simulink model "Model4"  (R2018b)
settings: Solver=VariableStepAuto  StartTime=0.0  StopTime=10.0  RelTol=1e-3
values from neighbouring files (symbols this model uses):
  P = 0    [Model.m]
undefined symbols (not defined in the file or in its folder): Ts
settings Model: Creator=Fabi Kadir  LastModifiedBy=Fabi Kadir

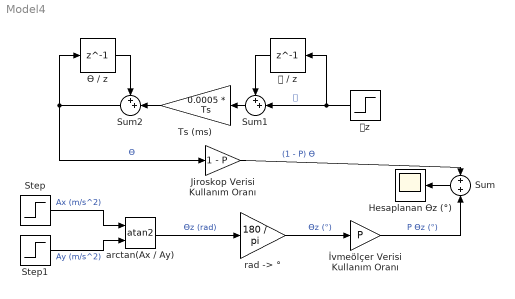
== system Model4 ==
  Hesaplanan Өz (°) : Scope
  Jiroskop Verisi Kullanım Oranı : Gain  Gain=1 - P
  Step : Step  SampleTime=0
  Step1 : Step  SampleTime=0
  Sum : Sum  Inputs=+|+
  Sum1 : Sum  Inputs=++|
  Sum2 : Sum  Inputs=++|
  Ts (ms) : Gain  Gain=0.0005 * Ts
  arctan(Ax / Ay) : Trigonometry  Operator=atan2
  "rad -> °" : Gain  Gain=180 / pi
  İvmeölçer Verisi Kullanım Oranı : Gain  Gain=P
  Ө / z : Delay  DelayLength=1
  Ꞷ / z : Delay  DelayLength=1
  Ꞷz : Step  SampleTime=0
  wires:
  Step/1 -> arctan(Ax / Ay)/1  "Ax (m/s^2)"
  arctan(Ax / Ay)/1 -> "rad -> °"/1  "Өz (rad)"
  Step1/1 -> arctan(Ax / Ay)/2  "Ay (m/s^2)"
  Sum/1 -> Hesaplanan Өz (°)/1
  Jiroskop Verisi Kullanım Oranı/1 -> Sum/1  "(1 - P) Ө"
  "rad -> °"/1 -> İvmeölçer Verisi Kullanım Oranı/1  "Өz (°)"
  İvmeölçer Verisi Kullanım Oranı/1 -> Sum/2  "P Өz (°)"
  Ꞷz/1 -> Sum1/2, Ꞷ / z/1  "Ꞷ"
  Ꞷ / z/1 -> Sum1/1
  Sum1/1 -> Ts (ms)/1
  Ts (ms)/1 -> Sum2/2
  Ө / z/1 -> Sum2/1
  Sum2/1 -> Jiroskop Verisi Kullanım Oranı/1, Ө / z/1  "Ө"
